simulink model "sfcndemo_sfun_errhdl"  (Simulink 6.0)
settings: Solver=FixedStepDiscrete  StartTime=0.0  StopTime=10.0  RelTol=1e-3
settings Model: Creator=The MathWorks Inc.  LastModifiedBy=batserve  ExtModeTrigMode=oneshot  ExtModeArmWhenConnect=off  ExtModeAutoUpdateStatusClock=off
settings DataIOCC: LimitDataPoints=off
settings OptimizationCC: BooleanDataType=off
settings DebuggingCC: CheckExecutionContextPreStartOutputMsg=on  CheckExecutionContextRuntimeOutputMsg=on  SolverPrmCheckMsg=none
settings HardwareCC: TargetUnknown=on

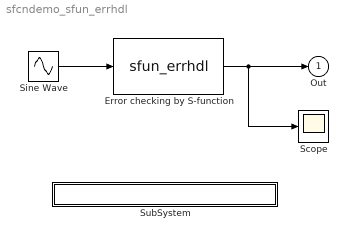
== system sfcndemo_sfun_errhdl ==
  Error checking by S-function : S-Function  FunctionName=sfun_errhdl  Parameters=param  mask(S-function: sfun_errhdl){param=2.3}
      mask prompts: param "Input parameter:"
      mask help: An example of handling parameter checking in S-function.
      mask Display: disp('Error\nHandling');
  Scope : Scope
      settings: TickLabels=on  TimeRange=10  YMin=-3  YMax=3  DataFormat=Array
  Sine Wave : Sin  SampleTime=0
  SubSystem : Subsystem  PropExecContextAcrossSSBoundary=on
      settings: OpenFcn=edit(fullfile(matlabroot,'simulink','src','sfun_errhdl.c'))
      mask Display: disp('matlabroot\simulink\src\sfun_errhdl.c');
  Out : Outport  InitialOutput=0
  wires:
  Sine Wave/1 -> Error checking by S-function/1
  Error checking by S-function/1 -> Out/1, Scope/1

== system sfcndemo_sfun_errhdl/SubSystem ==
